simulink model "dspanc_fixpt"  (Simulink 8.3)
settings: Solver=FixedStepDiscrete  StartTime=0.0  StopTime=inf  RelTol=1e-3
undefined symbols (not defined in the file or in its folder): dfilt
libraries: dspsrcs4 x2, dspsnks4 x2, dsparch4 x1, dspsigops x1, dspmisc x1, dspadpt3 x1
CloseFcn:
  | clear y_noisy;
  | clear y_org;
settings Model: Creator=The MathWorks Inc.  ExtModeAutoUpdateStatusClock=off
settings DataIOCC: LimitDataPoints=off  SaveOutput=off  SaveTime=off  SignalLoggingName=sigsOut
settings OptimizationCC: ExpressionDepthLimit=2147483647  InitFltsAndDblsToZero=on  EfficientMapNaN2IntZero=off
settings DebuggingCC: CheckExecutionContextPreStartOutputMsg=on  CheckExecutionContextRuntimeOutputMsg=on  SignalResolutionControl=TryResolveAllWithWarning  SolverPrmCheckMsg=none  MultiTaskDSMMsg=warning  MultiTaskCondExecSysMsg=none  IntegerOverflowMsg=none  ParameterPrecisionLossMsg=none  FcnCallInpInsideContextMsg=UseLocalSettings
settings HardwareCC: TargetUnknown=on
settings ModelReferenceCC: UpdateModelReferenceTargets=IfOutOfDate
settings RTWCC: IncludeERTFirstTime=on
settings GRTTargetCC: TargetFcnLib=ansi_tfl_tmw_new.mat

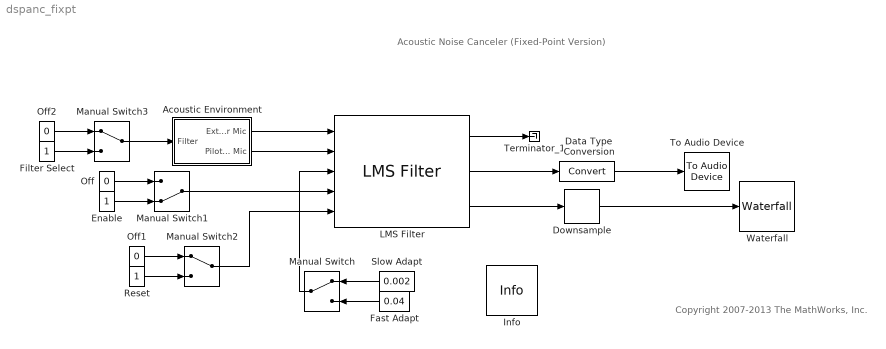
== system dspanc_fixpt ==
  note: Acoustic Noise Canceler (Fixed-Point Version)
  note: Copyright 2007-2013 The MathWorks, Inc.
  Acoustic Environment : Subsystem
  Data Type  Conversion : DataTypeConversion  SaturateOnIntegerOverflow=on  RndMeth=Zero
  Downsample : dspsigops/Downsample  N=32  phase=0  RateOptions=Allow multirate processing  smode=Allow multirate  fmode=Maintain input frame size  ic=0
  Enable : Constant  OutDataTypeStr=boolean
  Fast Adapt : Constant  Value=0.04  OutDataTypeStr=fixdt(1,16,15)
  Filter Select : Constant  OutDataTypeStr=boolean
  Info : dspmisc/Info  SystemSampleTime=-1
  LMS Filter : dspadpt3/LMS Filter  Algo=Normalized LMS  L=40  stepflag=Input port  mu=0.1  leakage=1.0  ic=0  Adapt=on  resetflag=Non-zero sample  weights=on  firstCoeffMode=Binary point scaling  firstCoeffWordLength=16  firstCoeffFracLength=16  secondCoeffMode=User-defined  secondCoeffWordLength=2  secondCoeffFracLength=14  accumMode=Binary point scaling  accumWordLength=32  accumFracLength=20  accum2Mode=User-defined  accum2FracLength=20  prodOutputMode=Binary point scaling  prodOutputWordLength=32  prodOutputFracLength=20  memoryMode=Binary point scaling  memoryWordLength=16  memoryFracLength=17  roundingMode=Nearest  overflowMode=on  addnparflag=off
  Manual Switch : ManualSwitch
  Manual Switch1 : ManualSwitch  CurrentSetting=0
  Manual Switch2 : ManualSwitch
  Manual Switch3 : ManualSwitch
  Off : Constant  Value=0  OutDataTypeStr=boolean
  Off1 : Constant  Value=0  OutDataTypeStr=boolean
  Off2 : Constant  Value=0  OutDataTypeStr=boolean
  Reset : Constant  OutDataTypeStr=boolean
  Slow Adapt : Constant  Value=0.002  OutDataTypeStr=fixdt(1,16,15)
  Terminator_1 : Terminator
  To Audio Device : dspsnks4/To Audio Device  deviceName=Default  inheritSampleRate=on  sampleRate=44100  deviceDatatype=Determine from input data type  autoBufferSize=on  bufferSize=4096  queueDuration=1  defaultOutputChannelMapping=on  outputChannelMapping=1:128
  Waterfall : dspsnks4/Waterfall  TraceProperties=on  NumTraces=6  CMapStr=autumn  TNewest=0.9  TOldest=0.5  HistoryLength=50  HistoryFull=Overwrite  UpdateInterval=1  ExportMode=All visible  MLExportName=ExportData  AutoExport=off  DisplayProperties=off  MouseMode=Orbit  AxisGrid=on  Snapshot=off  Suspend=off  SyncSnapshots=off  OpenScopeAtSimStart=on  FigPos=[27 57 405 339]  CameraView=[28.5695107359948 1316.8235109177 -294.350451091202 -0.004386576265097 22.5 3.5 0.594111941595966 -49.3321641526923 11.3523452384532 1.12783221137103 1 122.332173767783 16.310956502371]  InportDimsHint=[40 1]  AxisProperties=off  AxisColor='w'  XLabel=Samples  YLabel=Amplitude  ZLabel=Time  TriggerProperties=off  TrigStartMode=Immediately  TrigStartT=0  TrigStartN=0  TrigStartFcn=trigbegin  TrigStopMode=Never  TrigStopT=0.1  TrigStopN=1  TrigStopFcn=trigend  TrigRearmMode=Never  TrigRearmT=0  TrigRearmN=0  TrigRearmFcn=trigrearm  XformProperties=off  XformMode=None  XformFcn=abs  XformExpr=(u+1)/2
      settings: YMin=-0.188312025368214  YMax=0.24
  wires:
  Downsample/1 -> Waterfall/1
  Acoustic Environment/1(Exterior Mic) -> LMS Filter/1
  Slow Adapt/1 -> Manual Switch/1
  Fast Adapt/1 -> Manual Switch/2
  Manual Switch/1 -> LMS Filter/3
  LMS Filter/3 -> Downsample/1
  Acoustic Environment/2(Pilot's Mic) -> LMS Filter/2
  LMS Filter/2 -> Data Type  Conversion/1
  LMS Filter/1 -> Terminator_1/1
  Off/1 -> Manual Switch1/1
  Enable/1 -> Manual Switch1/2
  Off1/1 -> Manual Switch2/1
  Reset/1 -> Manual Switch2/2
  Manual Switch1/1 -> LMS Filter/4
  Manual Switch2/1 -> LMS Filter/5
  Off2/1 -> Manual Switch3/1
  Filter Select/1 -> Manual Switch3/2
  Manual Switch3/1 -> Acoustic Environment/1(Filter)
  Data Type  Conversion/1 -> To Audio Device/1

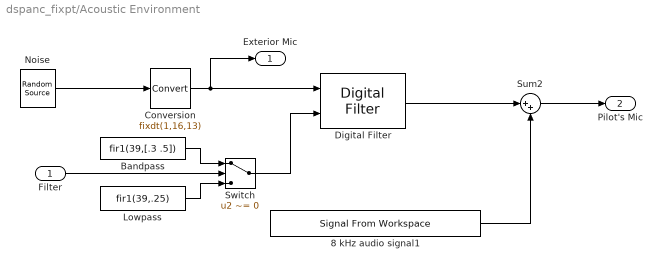
== system dspanc_fixpt/Acoustic Environment ==
  Filter : Inport
  8 kHz audio signal1 : dspsrcs4/Signal From Workspace  X=fi(audioread('dspafxf_8000.wav'),1,16,15)  Ts=1/8000  nsamps=32  OutputAfterFinalValue=Cyclic repetition  ignoreOrWarnInputAndFrameLengths=off
  Bandpass : Constant  Value=fir1(39,[.3 .5])  OutDataTypeStr=fixdt(1,16,17)
  Conversion : DataTypeConversion  OutDataTypeStr=fixdt(1,16,13)  RndMeth=Nearest
  Digital Filter : dsparch4/Digital Filter  TypePopup=FIR (all zeros)  IIRFiltStruct=Direct form II transposed  AllPoleFiltStruct=Direct form  FIRFiltStruct=Direct form  CoeffSource=Input port(s)  NumCoeffs=[1 2]  DenCoeffs=[1 0.1]  BiQuadCoeffs=[1 0.3 0.4 1 0.1 0.2]  LatticeCoeffs=[0.2 0.4]  denIgnore=on  FiltPerSampPopup=One filter per frame  IC=0  ICnum=0  ICden=0  accumMode=Binary point scaling  accumWordLength=32  accumFracLength=30  prodOutputMode=Binary point scaling  prodOutputWordLength=32  prodOutputFracLength=30  roundingMode=Nearest  overflowMode=off  ScaleValues=0  scaleValueFracLength=14  stageInFracLength=15  stageOutFracLength=15  FilterSource=Input port(s)  dfiltObjectName=dfilt.dffir([1 2 1])  InputProcessing=Columns as channels (frame based)
      settings: additionalParams=on  showOut=on  showAcc=on  showMpy=on
  Lowpass : Constant  Value=fir1(39,.25)  OutDataTypeStr=fixdt(1,16,17)
  Noise : dspsrcs4/Random Source  SrcType=Gaussian  NormMethod=Sum of uniform values  CltLength=5  MinVal=-1  MaxVal=1  MeanVal=0  VarVal=1  RepMode=Specify seed  rawSeed=[23342]  IsInherit=off  SampMode=Discrete  SampTime=1/8000  SampFrame=32  DataType=Single  OutComplex=Real
  Sum2 : Sum  Inputs=|++  RndMeth=Nearest  SaturateOnIntegerOverflow=on  OutDataTypeStr=Inherit: Same as first input
  Switch : Switch  Criteria=u2 ~= 0  SaturateOnIntegerOverflow=on
  Exterior Mic : Outport
  Pilot's Mic : Outport  Port=2
  wires:
  Noise/1 -> Conversion/1
  Conversion/1 -> Exterior Mic/1, Digital Filter/1
  Lowpass/1 -> Switch/3
  Bandpass/1 -> Switch/1
  Switch/1 -> Digital Filter/2
  Digital Filter/1 -> Sum2/1
  Filter/1 -> Switch/2
  Sum2/1 -> Pilot's Mic/1
  8 kHz audio signal1/1 -> Sum2/2
